simulink model "example_Storage_type3"  (R2018b)
settings: Solver=ode45  StartTime=0.0  StopTime=3*3600-2  RelTol=1e-3  EnableMultiTasking=on
undefined symbols (not defined in the file): path_carnot
libraries: carnot x12, simulink x3
settings Model: Creator=drhf  LastModifiedBy=P41573
settings DataIOCC: LimitDataPoints=on  SaveFormat=Array
settings OptimizationCC: ExpressionDepthLimit=2147483647  LifeSpan=inf
settings DebuggingCC: UnderspecifiedInitializationDetection=Classic  MergeDetectMultiDrivingBlocksExec=none  SolverPrmCheckMsg=warning  StateNameClashWarn=warning  SFUnexpectedBacktrackingDiag=warning  SFNoUnconditionalDefaultTransitionDiag=warning  SFExecutionAtInitializationDiag=none
settings HardwareCC: ProdBitPerPointer=32  ProdBitPerSizeT=32  ProdBitPerPtrDiffT=32  ProdLargestAtomicFloat=None  ProdIntDivRoundTo=Undefined  ProdEndianess=Unspecified  ProdWordSize=32  ProdHWDeviceType=32-bit Generic
settings ModelReferenceCC: PropagateSignalLabelsOutOfModel=off
settings SFSimCC: SimUseLocalCustomCode=off
settings RTWCC: RTWUseLocalCustomCode=off
settings CodeAppCC: StateflowObjectComments=on
settings GRTTargetCC: TargetLangStandard=C89/C90 (ANSI)  GeneratePreprocessorConditionals=Disable all  CombineOutputUpdateFcns=off  GRTInterface=on
settings ConfigComp: CovMetricSettings=dw  CovHtmlReporting=on  CovSaveCumulativeToWorkspaceVar=on  CovSaveSingleToWorkspaceVar=on  CovExternalEMLEnable=off

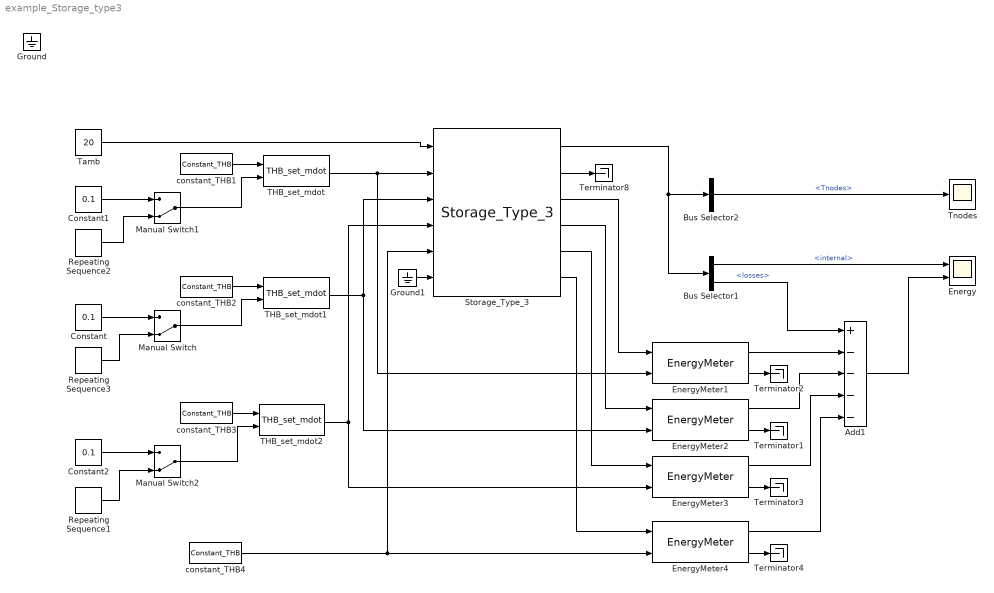
== system example_Storage_type3 ==
  Add1 : Sum  Inputs=+----
  Bus Selector1 : BusSelector  OutputSignals=energy.internal,energy.losses
  Bus Selector2 : BusSelector  OutputSignals=Tnodes
  Constant : Constant  Value=0.1
  Constant1 : Constant  Value=0.1
  Constant2 : Constant  Value=0.1
  Energy : Scope  NumInputPorts=2
  EnergyMeter{1..4} (4 alike) : carnot/Control/EnergyMeter
      settings: SourceProductName=Carnot
  Ground : Ground
  Ground1 : Ground
  Manual Switch : ManualSwitch  CurrentSetting=0
  Manual Switch1 : ManualSwitch  CurrentSetting=0
  Manual Switch2 : ManualSwitch  CurrentSetting=0
  Repeating Sequence1 : simulink/Sources/Repeating Sequence  rep_seq_t=[ 0 3600 3600+eps(3600) 7200 7200+eps(7200) 10800]  rep_seq_y=[ 0.12 0.12 0.11+0*eps(3600) 0.11 0.05+0*eps(7200) 0.05]
  Repeating Sequence2 : simulink/Sources/Repeating Sequence  rep_seq_t=[ 0 3600 3600+eps(3600) 7200 7200+eps(7200) 10440 10440+eps(10440) 11160]  rep_seq_y=[ 0 0 0.05+0*eps(3600) 0.05 0.2+0*eps(7200) 0.2 0+0*eps(10440) 0]
  Repeating Sequence3 : simulink/Sources/Repeating Sequence  rep_seq_t=[ 0 3600 3600+eps(3600) 7200 7200+eps(7200) 10800]  rep_seq_y=[ 0 0 0.1+0*eps(3600) 0.1 0.15+0*eps(7200) 0.15]
  Storage_Type_3 : carnot/Storage/Thermal/Storage_Type_3  t0=[10:5:55]  hgt=1.5279  stgtype=3  tini=[10 15 20 25 30 35 40 45 50 55]  mpts=[1 2 3 4 5 6 7 8 9 10]  PathName=fullfile(path_carnot('libsl'),'Storage','Thermal','Storage_Type_3','parameter_set')  FileName='StorageType3_300_L.mat'  userPath=off  userParam=off  uwall=1  ubot=1  utop=1  axcond=1  volume=0.3  dia=0.5  standing=standing cylinder  nodes=10  mpoints=10  Tsensor=[0.1 0.5 0.7]  hx1inlet=0.8  hx1outlet=0.6  hx1dia=0.03  hx1uac=50  hx1uam=0.15  hx1uat=0.6  hx1_uat2=0  hx1dpqua=20  hx1dplin=20  hx2inlet=0.4  hx2outlet=0  hx2dia=0.03  hx2uac=100  hx2uam=0.15  hx2uat=0.6  hx2_uat2=0  hx2dplin=30  hx2dpqua=30  pipe1inlet=0  pipe1outlet=1  pipe1dia=0.03  pipe2inlet=0.6  pipe2outlet=1  pipe2dia=0.03  heater1start=0.6  heater1end=0.65
      settings: SourceProductName=Carnot
  THB_set_mdot : carnot/Source/Simple/THB_set_mdot
      settings: SourceProductName=Carnot
  THB_set_mdot1 : carnot/Source/Simple/THB_set_mdot
      settings: SourceProductName=Carnot
  THB_set_mdot2 : carnot/Source/Simple/THB_set_mdot
      settings: SourceProductName=Carnot
  Tamb : Constant  Value=20
  Terminator{1..4,8} (5 alike) : Terminator
  Tnodes : Scope
  constant_THB1 : carnot/Source/Simple/Constant_THB  t=10  mdot=0*100/3600  p=1e5  mID=Full Pressure Drop with Static Height  fluid=Water  mix=0  mix2=0  mix3=0  dia=0.02  hgt=0
      settings: SourceProductName=Carnot
  constant_THB2 : carnot/Source/Simple/Constant_THB  t=55  mdot=0*100/3600  p=1e5  mID=Full Pressure Drop with Static Height  fluid=Water  mix=0  mix2=0  mix3=0  dia=0.02  hgt=0
      settings: SourceProductName=Carnot
  constant_THB3 : carnot/Source/Simple/Constant_THB  t=35  mdot=0*100/3600  p=1e5  mID=Full Pressure Drop with Static Height  fluid=Water  mix=0  mix2=0  mix3=0  dia=0.02  hgt=0
      settings: SourceProductName=Carnot
  constant_THB4 : carnot/Source/Simple/Constant_THB  t=35  mdot=0  p=1e5  mID=Full Pressure Drop with Static Height  fluid=Water  mix=0  mix2=0  mix3=0  dia=0.02  hgt=0
      settings: SourceProductName=Carnot
  wires:
  Tamb/1 -> Storage_Type_3/1
  THB_set_mdot/1 -> EnergyMeter1/2, Storage_Type_3/2
  THB_set_mdot1/1 -> Storage_Type_3/3, EnergyMeter2/2
  Storage_Type_3/1 -> Bus Selector1/1, Bus Selector2/1
  EnergyMeter2/2 -> Terminator1/1
  Manual Switch1/1 -> THB_set_mdot/2
  Manual Switch/1 -> THB_set_mdot1/2
  Constant/1 -> Manual Switch/1
  Repeating Sequence3/1 -> Manual Switch/2
  Constant1/1 -> Manual Switch1/1
  Repeating Sequence2/1 -> Manual Switch1/2
  EnergyMeter1/2 -> Terminator2/1
  EnergyMeter2/1 -> Add1/3
  EnergyMeter1/1 -> Add1/2
  Manual Switch2/1 -> THB_set_mdot2/2
  Constant2/1 -> Manual Switch2/1
  Repeating Sequence1/1 -> Manual Switch2/2
  THB_set_mdot2/1 -> EnergyMeter3/2, Storage_Type_3/4
  Storage_Type_3/2 -> Terminator8/1
  EnergyMeter3/2 -> Terminator3/1
  EnergyMeter3/1 -> Add1/4
  constant_THB1/1 -> THB_set_mdot/1
  constant_THB2/1 -> THB_set_mdot1/1
  constant_THB3/1 -> THB_set_mdot2/1
  Bus Selector1/1 -> Energy/1  "<internal>"
  Bus Selector2/1 -> Tnodes/1  "<Tnodes>"
  constant_THB4/1 -> Storage_Type_3/5, EnergyMeter4/2
  Bus Selector1/2 -> Add1/1  "<losses>"
  EnergyMeter4/2 -> Terminator4/1
  Storage_Type_3/3 -> EnergyMeter1/1
  EnergyMeter4/1 -> Add1/5
  Storage_Type_3/4 -> EnergyMeter2/1
  Storage_Type_3/5 -> EnergyMeter3/1
  Storage_Type_3/6 -> EnergyMeter4/1
  Add1/1 -> Energy/2
  Ground1/1 -> Storage_Type_3/6
